simulink model "Walsh_CDMA"  (Simulink 8.1)
settings: Solver=ode45  StartTime=0.0  StopTime=10.0  RelTol=1e-3
libraries: commutil2 x8, commseqgen2 x4, commfilt2 x2, commrandsrc2 x2
settings Model: Creator=mrinal  LastModifiedBy=Karan
settings DebuggingCC: FcnCallInpInsideContextMsg=EnableAllAsWarning
settings ConfigurationSet: Description=SimMechanics 2G

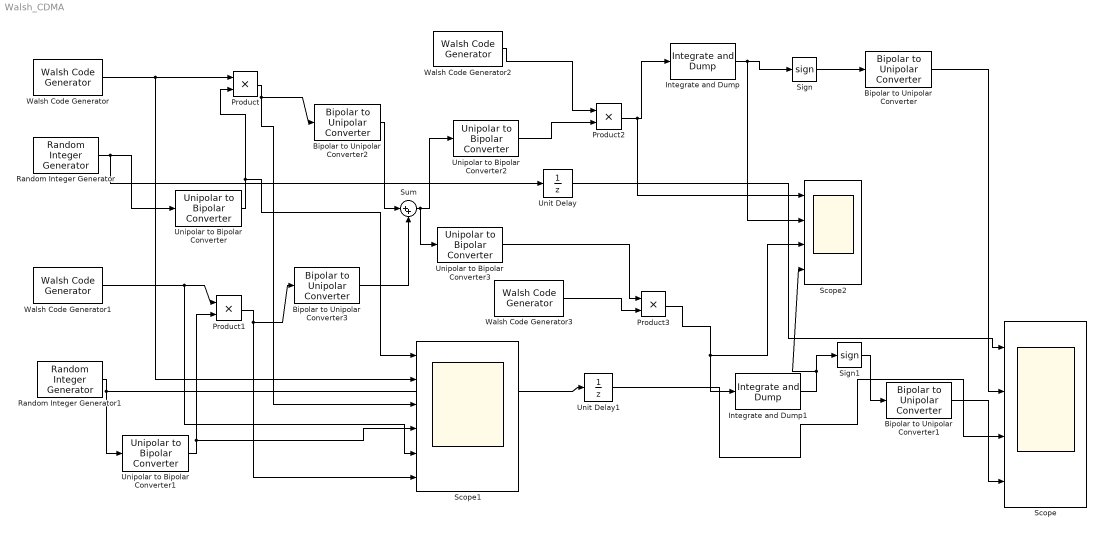
== system Walsh_CDMA ==
  Bipolar to Unipolar Converter{,1..3} (4 alike) : commutil2/Bipolar to Unipolar Converter  M=2  polarity=Positive  dataType=Inherit via internal rule
  Integrate and Dump : commfilt2/Integrate and Dump  obssamples=10  offsetsamples=0  nodump=off  roundingMode=Floor  overflowMode=off
  Integrate and Dump1 : commfilt2/Integrate and Dump  obssamples=10  offsetsamples=0  nodump=off  roundingMode=Floor  overflowMode=off
  Product{,1..3} (4 alike) : Product  RndMeth=Zero
  Random Integer Generator : commrandsrc2/Random Integer Generator  mul=2  seed=37  Ts=1  frameBased=off  sampPerFrame=1  orient=off  outDataType=double
  Random Integer Generator1 : commrandsrc2/Random Integer Generator  mul=2  seed=40  Ts=1  frameBased=off  sampPerFrame=1  orient=off  outDataType=double
  Scope : Scope  NumInputPorts=4
      settings: YMin=-5~-5~-5~-5  YMax=5~5~5~5  SampleInput=on  SampleTime=1
  Scope1 : Scope  NumInputPorts=6
      settings: YMin=-5~-5~-5~-5~-5~-5  YMax=5~5~5~5~5~5
  Scope2 : Scope  NumInputPorts=4
      settings: YMin=-5~-5~-5~-5  YMax=5~5~5~5  SaveName=ScopeData2
  Sign : Signum
  Sign1 : Signum
  Sum : Sum  Inputs=|++
  Unipolar to Bipolar Converter{,1..3} (4 alike) : commutil2/Unipolar to Bipolar Converter  M=2  polarity=Positive  dataType=Inherit via internal rule
  Unit Delay : UnitDelay  SampleTime=-1
  Unit Delay1 : UnitDelay  SampleTime=-1
  Walsh Code Generator : commseqgen2/Walsh Code Generator  length=64  index=60  ts=.1  frameBased=off  sampPerFrame=10  outDataType=double
  Walsh Code Generator1 : commseqgen2/Walsh Code Generator  length=64  index=55  ts=.1  frameBased=off  sampPerFrame=10  outDataType=double
  Walsh Code Generator2 : commseqgen2/Walsh Code Generator  length=64  index=60  ts=.1  frameBased=off  sampPerFrame=10  outDataType=double
  Walsh Code Generator3 : commseqgen2/Walsh Code Generator  length=64  index=55  ts=.1  frameBased=off  sampPerFrame=10  outDataType=double
  wires:
  Walsh Code Generator/1 -> Product/1, Scope1/2
  Walsh Code Generator2/1 -> Product2/1
  Product/1 -> Scope1/3, Bipolar to Unipolar Converter2/1
  Random Integer Generator/1 -> Unipolar to Bipolar Converter/1, Unit Delay/1
  Unipolar to Bipolar Converter/1 -> Product/2, Scope1/1
  Walsh Code Generator1/1 -> Product1/1, Scope1/5
  Random Integer Generator1/1 -> Unit Delay1/1, Unipolar to Bipolar Converter1/1
  Unipolar to Bipolar Converter1/1 -> Product1/2, Scope1/4
  Product1/1 -> Scope1/6, Bipolar to Unipolar Converter3/1
  Walsh Code Generator3/1 -> Product3/2
  Product2/1 -> Integrate and Dump/1, Scope2/1
  Product3/1 -> Integrate and Dump1/1, Scope2/3
  Integrate and Dump/1 -> Scope2/2, Sign/1
  Integrate and Dump1/1 -> Sign1/1, Scope2/4
  Sign/1 -> Bipolar to Unipolar Converter/1
  Sign1/1 -> Bipolar to Unipolar Converter1/1
  Bipolar to Unipolar Converter2/1 -> Sum/1
  Bipolar to Unipolar Converter3/1 -> Sum/2
  Sum/1 -> Unipolar to Bipolar Converter2/1, Unipolar to Bipolar Converter3/1
  Unipolar to Bipolar Converter2/1 -> Product2/2
  Unipolar to Bipolar Converter3/1 -> Product3/1
  Bipolar to Unipolar Converter/1 -> Scope/2
  Bipolar to Unipolar Converter1/1 -> Scope/4
  Unit Delay/1 -> Scope/1
  Unit Delay1/1 -> Scope/3
